simulink model "AltControl"  (R2024a)
settings: Solver=ode4  StartTime=0.0  StopTime=10.0  FixedStep=1/1200  RelTol=1e-3
undefined symbols (not defined in the file): DiscIntNeverNeededParam, wind_x, wind_y, wind_z
libraries: Sensors x2, PosControl x1, GT x1
settings Model: Creator=igmso  LastModifiedBy=igmso
settings DataIOCC: SaveFormat=StructureWithTime

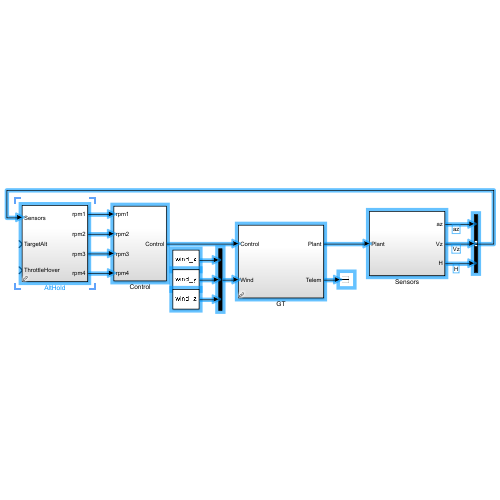
[thumbnail: Simulink's stored preview of the top-level diagram]
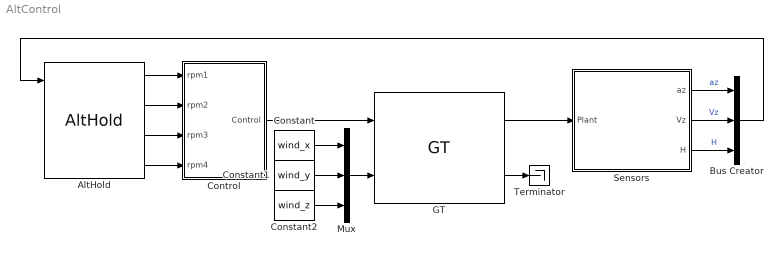
== system AltControl ==
  AltHold : PosControl/AltHold  SystemSampleTime=-1  VariantActivationTime=update diagram  AllowFlexibleInterface=on  Latency=0  AutoFrameSizeCalculation=off
  Bus Creator : BusCreator  Inputs=3
  Constant : Constant  Value=wind_x
  Constant1 : Constant  Value=wind_y
  Constant2 : Constant  Value=wind_z
  Control : Subsystem
  GT : GT/GT  SystemSampleTime=-1  VariantActivationTime=update diagram  AllowFlexibleInterface=on  Latency=0  AutoFrameSizeCalculation=off
  Mux : Mux  Inputs=3
  Sensors : Subsystem
  Terminator : Terminator
  wires:
  Constant/1 -> Mux/1
  Constant2/1 -> Mux/3
  Constant1/1 -> Mux/2
  Mux/1 -> GT/2
  GT/2 -> Terminator/1
  GT/1 -> Sensors/1(Plant)
  Control/1(Control) -> GT/1
  Sensors/2(Vz) -> Bus Creator/2  "Vz"
  Sensors/1(az) -> Bus Creator/1  "az"
  Sensors/3(H) -> Bus Creator/3  "H"
  Bus Creator/1 -> AltHold/1
  AltHold/4 -> Control/4(rpm4)
  AltHold/3 -> Control/3(rpm3)
  AltHold/2 -> Control/2(rpm2)
  AltHold/1 -> Control/1(rpm1)

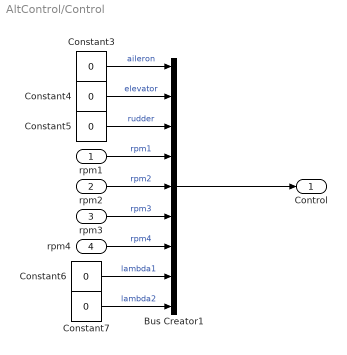
== system AltControl/Control ==
  rpm1 : Inport
  rpm2 : Inport  Port=2
  rpm3 : Inport  Port=3
  rpm4 : Inport  Port=4
  Bus Creator1 : BusCreator  Inputs=9
  Constant{3..7} (5 alike) : Constant  Value=0  SampleTime=-1
  Control : Outport
  wires:
  Constant4/1 -> Bus Creator1/2  "elevator"
  rpm3/1 -> Bus Creator1/6  "rpm3"
  Constant5/1 -> Bus Creator1/3  "rudder"
  Constant7/1 -> Bus Creator1/9  "lambda2"
  rpm4/1 -> Bus Creator1/7  "rpm4"
  Constant3/1 -> Bus Creator1/1  "aileron"
  Bus Creator1/1 -> Control/1
  Constant6/1 -> Bus Creator1/8  "lambda1"
  rpm1/1 -> Bus Creator1/4  "rpm1"
  rpm2/1 -> Bus Creator1/5  "rpm2"

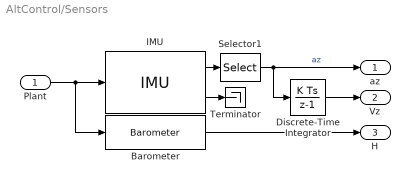
== system AltControl/Sensors ==
  Plant : Inport
  Barometer : Sensors/Barometer  SystemSampleTime=-1  VariantActivationTime=update diagram  AllowFlexibleInterface=on  Latency=0  AutoFrameSizeCalculation=off
  Discrete-Time Integrator : DiscreteIntegrator  SampleTime=1/400  StateName='Vz'  ICPrevOutput=DiscIntNeverNeededParam  ICPrevScaledInput=DiscIntNeverNeededParam
  IMU : Sensors/IMU  SystemSampleTime=-1  VariantActivationTime=update diagram  AllowFlexibleInterface=on  Latency=0  AutoFrameSizeCalculation=off
  Selector1 : Selector  InputPortWidth=3  IndexOptions=Index vector (dialog)  Indices=3  OutputSizes=1
  Terminator : Terminator
  az : Outport
  Vz : Outport  Port=2
  H : Outport  Port=3
  wires:
  Plant/1 -> Barometer/1, IMU/1
  Barometer/1 -> H/1
  IMU/2 -> Terminator/1
  IMU/1 -> Selector1/1
  Selector1/1 -> Discrete-Time Integrator/1, az/1  "az"
  Discrete-Time Integrator/1 -> Vz/1
